simulink library "halout"  (R2021b)
settings: Solver=VariableStepAuto  StartTime=0.0  StopTime=10.0  RelTol=1e-3
undefined symbols (not defined in the file): C_TASK_5MS_S, FALSE, KHAL_CAN1FD1APS3E2E_flg, KHAL_CAN1FD1APS3TxReq_flg, KHAL_CAN1FD1VCU2E2E_flg, KHAL_CAN1FD1VCU2TxReq_flg, KHAL_CAN1FD1VCU3E2E_flg, KHAL_CAN1FD1VCU3TxReq_flg, KHAL_CAN1TxReq_flg, KHAL_CAN1VMCFCM1E2E_flg, KHAL_CAN1VMCFCM1TxReq_flg, KHAL_CAN2TxReq_flg, KHAL_CAN3FD3VCU1toNIDECTxReq_flg, KHAL_CAN3FD3VCU1TxReq_flg, KHAL_CAN3FD3VCU2E2E_flg, KHAL_CAN3FD3VCU2toNIDECE2E_flg, KHAL_CAN3FD3VCU2toNIDECTxReq_flg, KHAL_CAN3FD3VCU2TxReq_flg, KHAL_CAN3TxReq_flg, KHAL_CAN4FD4CE1000E2E_flg, KHAL_CAN4FD4CE1000TxReq_flg, KHAL_CAN4TxReq_flg, KHAL_CAN5TxReq_flg, KHAL_CAN6FD6APS3E2E_flg, KHAL_CAN6FD6APS3TxReq_flg, KHAL_CAN6FD6VCU2E2E_flg, KHAL_CAN6FD6VCU2TxReq_flg, KHAL_CAN6TxReq_flg, ONE_INT, TRUE, ZERO_INT
libraries: FVT_lib x549, simulink x244
(part 17 of 27)

== system halout/HAL_OUT/CAN1/VMC_FCM1_0x172/Byte_13 ==
  FDC_VMC_AngCtrlTqWtGn : Inport
  BitwiseOR : simulink/Logic and Bit Operations/Bitwise Operator  logicop=OR  UseBitMask=off  BitMask=bin2dec('11011001')  BitMaskRealWorld=Stored Integer
  SignalPack : FVT_lib/hal/SignalPack  RightShiftCnt=0  BitMask=2^8-1  LeftShiftCnt=0
  UnitConverter : DataTypeConversion  OutDataTypeStr=uint8  RndMeth=Round
  UnitConverter1 : DataTypeConversion  OutDataTypeStr=uint8  RndMeth=Round
  convert_out : FVT_lib/hal/convert_out  gain=0.4  offset=0
  Byte_13 : Outport
  wires:
  BitwiseOR/1 -> Byte_13/1
  UnitConverter/1 -> BitwiseOR/1
  SignalPack/1 -> UnitConverter/1
  UnitConverter1/1 -> SignalPack/1
  convert_out/1 -> UnitConverter1/1
  FDC_VMC_AngCtrlTqWtGn/1 -> convert_out/1

== system halout/HAL_OUT/CAN1/VMC_FCM1_0x172/Byte_14 ==
  FDC_VMC_DrInpTqBstGn : Inport
  BitwiseOR : simulink/Logic and Bit Operations/Bitwise Operator  logicop=OR  UseBitMask=off  BitMask=bin2dec('11011001')  BitMaskRealWorld=Stored Integer
  SignalPack : FVT_lib/hal/SignalPack  RightShiftCnt=0  BitMask=2^8-1  LeftShiftCnt=0
  UnitConverter : DataTypeConversion  OutDataTypeStr=uint8  RndMeth=Round
  UnitConverter1 : DataTypeConversion  OutDataTypeStr=uint8  RndMeth=Round
  convert_out : FVT_lib/hal/convert_out  gain=0.4  offset=0
  Byte_14 : Outport
  wires:
  BitwiseOR/1 -> Byte_14/1
  UnitConverter/1 -> BitwiseOR/1
  SignalPack/1 -> UnitConverter/1
  UnitConverter1/1 -> SignalPack/1
  convert_out/1 -> UnitConverter1/1
  FDC_VMC_DrInpTqBstGn/1 -> convert_out/1

== system halout/HAL_OUT/CAN1/VMC_FCM1_0x172/Byte_15 ==
  FDC_VMC_DMSMode_Cmd : Inport
  BitwiseOR : simulink/Logic and Bit Operations/Bitwise Operator  logicop=OR  UseBitMask=off  BitMask=bin2dec('11011001')  BitMaskRealWorld=Stored Integer
  SignalPack : FVT_lib/hal/SignalPack  RightShiftCnt=0  BitMask=2^4-1  LeftShiftCnt=0
  UnitConverter : DataTypeConversion  OutDataTypeStr=uint8  RndMeth=Round
  UnitConverter1 : DataTypeConversion  OutDataTypeStr=uint8  RndMeth=Round
  Byte_15 : Outport
  wires:
  BitwiseOR/1 -> Byte_15/1
  UnitConverter/1 -> BitwiseOR/1
  SignalPack/1 -> UnitConverter/1
  UnitConverter1/1 -> SignalPack/1
  FDC_VMC_DMSMode_Cmd/1 -> UnitConverter1/1

== system halout/HAL_OUT/CAN1/VMC_FCM1_0x172/Byte_2 ==
  VMC_FCM_LKA_TOIAct : Inport
  BitwiseOR : simulink/Logic and Bit Operations/Bitwise Operator  logicop=OR  UseBitMask=off  BitMask=bin2dec('11011001')  BitMaskRealWorld=Stored Integer
  SignalPack : FVT_lib/hal/SignalPack  RightShiftCnt=0  BitMask=2^8-1  LeftShiftCnt=0
  UnitConverter : DataTypeConversion  OutDataTypeStr=uint8  RndMeth=Round
  UnitConverter1 : DataTypeConversion  OutDataTypeStr=uint8  RndMeth=Round
  Byte_2 : Outport
  wires:
  BitwiseOR/1 -> Byte_2/1
  UnitConverter/1 -> BitwiseOR/1
  SignalPack/1 -> UnitConverter/1
  UnitConverter1/1 -> SignalPack/1
  VMC_FCM_LKA_TOIAct/1 -> UnitConverter1/1

== system halout/HAL_OUT/CAN1/VMC_FCM1_0x172/Byte_3 ==
  VMC_AEB_VehHoldReq : Inport
  VMC_FCM_LDW_Fault : Inport  Port=2
  VMC_FCM_LDW_Request : Inport  Port=3
  VMC_FCM_LKA_StrToqReq : Inport  Port=4
  VMC_FCM_LKA_TOIFault : Inport  Port=5
  BitwiseOR : simulink/Logic and Bit Operations/Bitwise Operator  logicop=OR  UseBitMask=off  NumInputPorts=5  BitMask=bin2dec('11011001')  BitMaskRealWorld=Stored Integer
  SignalPack : FVT_lib/hal/SignalPack  RightShiftCnt=0  BitMask=2^1-1  LeftShiftCnt=3
  SignalPack1 : FVT_lib/hal/SignalPack  RightShiftCnt=0  BitMask=2^1-1  LeftShiftCnt=5
  SignalPack2 : FVT_lib/hal/SignalPack  RightShiftCnt=0  BitMask=2^2-1  LeftShiftCnt=6
  SignalPack3 : FVT_lib/hal/SignalPack  RightShiftCnt=8  BitMask=2^3-1  LeftShiftCnt=0
  SignalPack4 : FVT_lib/hal/SignalPack  RightShiftCnt=0  BitMask=2^1-1  LeftShiftCnt=4
  UnitConverter{,1..6,8..9} (9 alike) : DataTypeConversion  OutDataTypeStr=uint8  RndMeth=Round
  UnitConverter7 : DataTypeConversion  OutDataTypeStr=uint16  RndMeth=Round
  convert_out : FVT_lib/hal/convert_out  gain=0.008  offset=-8
  Byte_3 : Outport
  wires:
  BitwiseOR/1 -> Byte_3/1
  UnitConverter/1 -> BitwiseOR/1
  SignalPack/1 -> UnitConverter/1
  UnitConverter1/1 -> SignalPack/1
  VMC_AEB_VehHoldReq/1 -> UnitConverter1/1
  UnitConverter2/1 -> BitwiseOR/2
  SignalPack1/1 -> UnitConverter2/1
  UnitConverter3/1 -> SignalPack1/1
  VMC_FCM_LDW_Fault/1 -> UnitConverter3/1
  UnitConverter4/1 -> BitwiseOR/3
  SignalPack2/1 -> UnitConverter4/1
  UnitConverter5/1 -> SignalPack2/1
  VMC_FCM_LDW_Request/1 -> UnitConverter5/1
  UnitConverter6/1 -> BitwiseOR/4
  SignalPack3/1 -> UnitConverter6/1
  UnitConverter7/1 -> SignalPack3/1
  convert_out/1 -> UnitConverter7/1
  VMC_FCM_LKA_StrToqReq/1 -> convert_out/1
  UnitConverter8/1 -> BitwiseOR/5
  SignalPack4/1 -> UnitConverter8/1
  UnitConverter9/1 -> SignalPack4/1
  VMC_FCM_LKA_TOIFault/1 -> UnitConverter9/1

== system halout/HAL_OUT/CAN1/VMC_FCM1_0x172/Byte_4 ==
  VMC_FCM_LKA_StrToqReq : Inport
  BitwiseOR : simulink/Logic and Bit Operations/Bitwise Operator  logicop=OR  UseBitMask=off  BitMask=bin2dec('11011001')  BitMaskRealWorld=Stored Integer
  SignalPack : FVT_lib/hal/SignalPack  RightShiftCnt=0  BitMask=2^8-1  LeftShiftCnt=0
  UnitConverter : DataTypeConversion  OutDataTypeStr=uint8  RndMeth=Round
  UnitConverter1 : DataTypeConversion  OutDataTypeStr=uint16  RndMeth=Round
  convert_out : FVT_lib/hal/convert_out  gain=0.008  offset=-8
  Byte_4 : Outport
  wires:
  BitwiseOR/1 -> Byte_4/1
  UnitConverter/1 -> BitwiseOR/1
  SignalPack/1 -> UnitConverter/1
  UnitConverter1/1 -> SignalPack/1
  convert_out/1 -> UnitConverter1/1
  VMC_FCM_LKA_StrToqReq/1 -> convert_out/1

== system halout/HAL_OUT/CAN1/VMC_FCM1_0x172/Byte_5 ==
  VMC_ACC_RequiredAccel : Inport
  VMC_ACC_VehHoldReq : Inport  Port=2
  VMC_ADAS_AEBReq : Inport  Port=3
  VMC_ADAS_DBSReq : Inport  Port=4
  VMC_ADAS_FaultSta : Inport  Port=5
  BitwiseOR : simulink/Logic and Bit Operations/Bitwise Operator  logicop=OR  UseBitMask=off  NumInputPorts=5  BitMask=bin2dec('11011001')  BitMaskRealWorld=Stored Integer
  SignalPack : FVT_lib/hal/SignalPack  RightShiftCnt=8  BitMask=2^1-1  LeftShiftCnt=0
  SignalPack1 : FVT_lib/hal/SignalPack  RightShiftCnt=0  BitMask=2^1-1  LeftShiftCnt=7
  SignalPack2 : FVT_lib/hal/SignalPack  RightShiftCnt=0  BitMask=2^3-1  LeftShiftCnt=1
  SignalPack3 : FVT_lib/hal/SignalPack  RightShiftCnt=0  BitMask=2^2-1  LeftShiftCnt=5
  SignalPack4 : FVT_lib/hal/SignalPack  RightShiftCnt=0  BitMask=2^1-1  LeftShiftCnt=4
  UnitConverter{,2..9} (9 alike) : DataTypeConversion  OutDataTypeStr=uint8  RndMeth=Round
  UnitConverter1 : DataTypeConversion  OutDataTypeStr=uint16  RndMeth=Round
  convert_out : FVT_lib/hal/convert_out  gain=0.05  offset=-15
  Byte_5 : Outport
  wires:
  BitwiseOR/1 -> Byte_5/1
  UnitConverter/1 -> BitwiseOR/1
  SignalPack/1 -> UnitConverter/1
  UnitConverter1/1 -> SignalPack/1
  convert_out/1 -> UnitConverter1/1
  VMC_ACC_RequiredAccel/1 -> convert_out/1
  UnitConverter2/1 -> BitwiseOR/2
  SignalPack1/1 -> UnitConverter2/1
  UnitConverter3/1 -> SignalPack1/1
  VMC_ACC_VehHoldReq/1 -> UnitConverter3/1
  UnitConverter4/1 -> BitwiseOR/3
  SignalPack2/1 -> UnitConverter4/1
  UnitConverter5/1 -> SignalPack2/1
  VMC_ADAS_AEBReq/1 -> UnitConverter5/1
  UnitConverter6/1 -> BitwiseOR/4
  SignalPack3/1 -> UnitConverter6/1
  UnitConverter7/1 -> SignalPack3/1
  VMC_ADAS_DBSReq/1 -> UnitConverter7/1
  UnitConverter8/1 -> BitwiseOR/5
  SignalPack4/1 -> UnitConverter8/1
  UnitConverter9/1 -> SignalPack4/1
  VMC_ADAS_FaultSta/1 -> UnitConverter9/1

== system halout/HAL_OUT/CAN1/VMC_FCM1_0x172/Byte_6 ==
  VMC_ACC_RequiredAccel : Inport
  BitwiseOR : simulink/Logic and Bit Operations/Bitwise Operator  logicop=OR  UseBitMask=off  BitMask=bin2dec('11011001')  BitMaskRealWorld=Stored Integer
  SignalPack : FVT_lib/hal/SignalPack  RightShiftCnt=0  BitMask=2^8-1  LeftShiftCnt=0
  UnitConverter : DataTypeConversion  OutDataTypeStr=uint8  RndMeth=Round
  UnitConverter1 : DataTypeConversion  OutDataTypeStr=uint16  RndMeth=Round
  convert_out : FVT_lib/hal/convert_out  gain=0.05  offset=-15
  Byte_6 : Outport
  wires:
  BitwiseOR/1 -> Byte_6/1
  UnitConverter/1 -> BitwiseOR/1
  SignalPack/1 -> UnitConverter/1
  UnitConverter1/1 -> SignalPack/1
  convert_out/1 -> UnitConverter1/1
  VMC_ACC_RequiredAccel/1 -> convert_out/1

== system halout/HAL_OUT/CAN1/VMC_FCM1_0x172/Byte_7 ==
  VMC_ACC_ComfortBandUpper : Inport
  VMC_ACC_JerkUpperLInit : Inport  Port=2
  BitwiseOR : simulink/Logic and Bit Operations/Bitwise Operator  logicop=OR  UseBitMask=off  NumInputPorts=2  BitMask=bin2dec('11011001')  BitMaskRealWorld=Stored Integer
  SignalPack : FVT_lib/hal/SignalPack  RightShiftCnt=8  BitMask=2^1-1  LeftShiftCnt=0
  SignalPack1 : FVT_lib/hal/SignalPack  RightShiftCnt=0  BitMask=2^7-1  LeftShiftCnt=1
  UnitConverter : DataTypeConversion  OutDataTypeStr=uint8  RndMeth=Round
  UnitConverter1 : DataTypeConversion  OutDataTypeStr=uint16  RndMeth=Round
  UnitConverter2 : DataTypeConversion  OutDataTypeStr=uint8  RndMeth=Round
  UnitConverter3 : DataTypeConversion  OutDataTypeStr=uint8  RndMeth=Round
  convert_out : FVT_lib/hal/convert_out  gain=0.05  offset=-15
  convert_out1 : FVT_lib/hal/convert_out  gain=0.1  offset=-6
  Byte_7 : Outport
  wires:
  BitwiseOR/1 -> Byte_7/1
  UnitConverter/1 -> BitwiseOR/1
  SignalPack/1 -> UnitConverter/1
  UnitConverter1/1 -> SignalPack/1
  convert_out/1 -> UnitConverter1/1
  VMC_ACC_ComfortBandUpper/1 -> convert_out/1
  UnitConverter2/1 -> BitwiseOR/2
  SignalPack1/1 -> UnitConverter2/1
  UnitConverter3/1 -> SignalPack1/1
  convert_out1/1 -> UnitConverter3/1
  VMC_ACC_JerkUpperLInit/1 -> convert_out1/1

== system halout/HAL_OUT/CAN1/VMC_FCM1_0x172/Byte_8 ==
  VMC_ACC_ComfortBandUpper : Inport
  BitwiseOR : simulink/Logic and Bit Operations/Bitwise Operator  logicop=OR  UseBitMask=off  BitMask=bin2dec('11011001')  BitMaskRealWorld=Stored Integer
  SignalPack : FVT_lib/hal/SignalPack  RightShiftCnt=0  BitMask=2^8-1  LeftShiftCnt=0
  UnitConverter : DataTypeConversion  OutDataTypeStr=uint8  RndMeth=Round
  UnitConverter1 : DataTypeConversion  OutDataTypeStr=uint16  RndMeth=Round
  convert_out : FVT_lib/hal/convert_out  gain=0.05  offset=-15
  Byte_8 : Outport
  wires:
  BitwiseOR/1 -> Byte_8/1
  UnitConverter/1 -> BitwiseOR/1
  SignalPack/1 -> UnitConverter/1
  UnitConverter1/1 -> SignalPack/1
  convert_out/1 -> UnitConverter1/1
  VMC_ACC_ComfortBandUpper/1 -> convert_out/1

== system halout/HAL_OUT/CAN1/VMC_FCM1_0x172/Byte_9 ==
  VMC_ACC_ComfortBandLower : Inport
  VMC_ACC_JerkLowerLInit : Inport  Port=2
  BitwiseOR : simulink/Logic and Bit Operations/Bitwise Operator  logicop=OR  UseBitMask=off  NumInputPorts=2  BitMask=bin2dec('11011001')  BitMaskRealWorld=Stored Integer
  SignalPack : FVT_lib/hal/SignalPack  RightShiftCnt=8  BitMask=2^1-1  LeftShiftCnt=0
  SignalPack1 : FVT_lib/hal/SignalPack  RightShiftCnt=0  BitMask=2^7-1  LeftShiftCnt=1
  UnitConverter : DataTypeConversion  OutDataTypeStr=uint8  RndMeth=Round
  UnitConverter1 : DataTypeConversion  OutDataTypeStr=uint16  RndMeth=Round
  UnitConverter2 : DataTypeConversion  OutDataTypeStr=uint8  RndMeth=Round
  UnitConverter3 : DataTypeConversion  OutDataTypeStr=uint8  RndMeth=Round
  convert_out : FVT_lib/hal/convert_out  gain=0.05  offset=-15
  convert_out1 : FVT_lib/hal/convert_out  gain=0.1  offset=-6
  Byte_9 : Outport
  wires:
  BitwiseOR/1 -> Byte_9/1
  UnitConverter/1 -> BitwiseOR/1
  SignalPack/1 -> UnitConverter/1
  UnitConverter1/1 -> SignalPack/1
  convert_out/1 -> UnitConverter1/1
  VMC_ACC_ComfortBandLower/1 -> convert_out/1
  UnitConverter2/1 -> BitwiseOR/2
  SignalPack1/1 -> UnitConverter2/1
  UnitConverter3/1 -> SignalPack1/1
  convert_out1/1 -> UnitConverter3/1
  VMC_ACC_JerkLowerLInit/1 -> convert_out1/1

== system halout/HAL_OUT/CAN1/VMC_FCM1_0x172/CRC8_IfAction_Tx ==
  CAN_E2E_flg : Inport
  DataID1 : Inport  Port=2
  DataID2 : Inport  Port=3
  RawData : Inport  Port=4
  Data Type Conversion : DataTypeConversion  OutDataTypeStr=uint8
  If : If
  If Action Subsystem : Subsystem  TreatAsAtomicUnit=on
  If Action Subsystem1 : Subsystem  TreatAsAtomicUnit=on
  Merge : Merge
  CRC8 : Outport
  wires:
  If/2 -> If Action Subsystem/Action
  If/1 -> If Action Subsystem1/Action
  CAN_E2E_flg/1 -> [CAN_E2E_flg]
  DataID1/1 -> [DataID1]
  DataID2/1 -> [DataID2]
  RawData/1 -> [RawData]
  [CAN_E2E_flg] -> Data Type Conversion/1
  [DataID1] -> If Action Subsystem1/1(CAN_E2E_ID1)
  [DataID2] -> If Action Subsystem1/2(CAN_E2E_ID2)
  [RawData] -> If Action Subsystem1/3(Byte1)
  [RawData] -> If Action Subsystem/1(Byte1)
  If Action Subsystem1/1(CRC8_E2EResult) -> Merge/1
  If Action Subsystem/1(CRC8_Result) -> Merge/2
  Merge/1 -> CRC8/1
  Data Type Conversion/1 -> If/1

== system halout/HAL_OUT/CAN1/VMC_FCM1_0x172/FDCVMCAngCtrlTqWtGn ==
  FDCVMCAngCtrlTqWtGn : Inport
  Data Type Conversion : DataTypeConversion  OutDataTypeStr=uint8  RndMeth=Round
  convert_out : FVT_lib/hal/convert_out  gain=0.4  offset=0
  CAN1_FDC_VMC_AngCtrlTqWtGn : Outport
  wires:
  Data Type Conversion/1 -> CAN1_FDC_VMC_AngCtrlTqWtGn/1
  convert_out/1 -> Data Type Conversion/1
  FDCVMCAngCtrlTqWtGn/1 -> convert_out/1

== system halout/HAL_OUT/CAN1/VMC_FCM1_0x172/FDCVMCDMSModeCmd ==
  FDCVMCDMSModeCmd : Inport
  Data Type Conversion : DataTypeConversion  OutDataTypeStr=uint8  RndMeth=Round
  CAN1_FDC_VMC_DMSMode_Cmd : Outport
  wires:
  Data Type Conversion/1 -> CAN1_FDC_VMC_DMSMode_Cmd/1
  FDCVMCDMSModeCmd/1 -> Data Type Conversion/1

== system halout/HAL_OUT/CAN1/VMC_FCM1_0x172/FDCVMCDrInpTqBstAct ==
  FDCVMCDrInpTqBstAct : Inport
  Data Type Conversion : DataTypeConversion  OutDataTypeStr=uint8  RndMeth=Round
  CAN1_FDC_VMC_DrInpTqBstAct : Outport
  wires:
  Data Type Conversion/1 -> CAN1_FDC_VMC_DrInpTqBstAct/1
  FDCVMCDrInpTqBstAct/1 -> Data Type Conversion/1

== system halout/HAL_OUT/CAN1/VMC_FCM1_0x172/FDCVMCDrInpTqBstGn ==
  FDCVMCDrInpTqBstGn : Inport
  Data Type Conversion : DataTypeConversion  OutDataTypeStr=uint8  RndMeth=Round
  convert_out : FVT_lib/hal/convert_out  gain=0.4  offset=0
  CAN1_FDC_VMC_DrInpTqBstGn : Outport
  wires:
  Data Type Conversion/1 -> CAN1_FDC_VMC_DrInpTqBstGn/1
  convert_out/1 -> Data Type Conversion/1
  FDCVMCDrInpTqBstGn/1 -> convert_out/1

== system halout/HAL_OUT/CAN1/VMC_FCM1_0x172/FDCVMCMaxAngCtrlOutTqLim ==
  FDCVMCMaxAngCtrlOutTqLim : Inport
  Data Type Conversion : DataTypeConversion  OutDataTypeStr=uint16  RndMeth=Round
  convert_out : FVT_lib/hal/convert_out  gain=0.1  offset=0
  CAN1_FDC_VMC_MaxAngCtrlOutTqLim : Outport
  wires:
  Data Type Conversion/1 -> CAN1_FDC_VMC_MaxAngCtrlOutTqLim/1
  convert_out/1 -> Data Type Conversion/1
  FDCVMCMaxAngCtrlOutTqLim/1 -> convert_out/1

== system halout/HAL_OUT/CAN1/VMC_FCM1_0x172/VMCACCComfortBandLower ==
  VMCACCComfortBandLower : Inport
  Data Type Conversion : DataTypeConversion  OutDataTypeStr=uint16  RndMeth=Round
  convert_out : FVT_lib/hal/convert_out  gain=0.05  offset=-15
  CAN1_VMC_ACC_ComfortBandLower : Outport
  wires:
  Data Type Conversion/1 -> CAN1_VMC_ACC_ComfortBandLower/1
  convert_out/1 -> Data Type Conversion/1
  VMCACCComfortBandLower/1 -> convert_out/1

== system halout/HAL_OUT/CAN1/VMC_FCM1_0x172/VMCACCComfortBandUpper ==
  VMCACCComfortBandUpper : Inport
  Data Type Conversion : DataTypeConversion  OutDataTypeStr=uint16  RndMeth=Round
  convert_out : FVT_lib/hal/convert_out  gain=0.05  offset=-15
  CAN1_VMC_ACC_ComfortBandUpper : Outport
  wires:
  Data Type Conversion/1 -> CAN1_VMC_ACC_ComfortBandUpper/1
  convert_out/1 -> Data Type Conversion/1
  VMCACCComfortBandUpper/1 -> convert_out/1

== system halout/HAL_OUT/CAN1/VMC_FCM1_0x172/VMCACCJerkLowerLInit ==
  VMCACCJerkLowerLInit : Inport
  Data Type Conversion : DataTypeConversion  OutDataTypeStr=uint8  RndMeth=Round
  convert_out : FVT_lib/hal/convert_out  gain=0.1  offset=-6
  CAN1_VMC_ACC_JerkLowerLInit : Outport
  wires:
  Data Type Conversion/1 -> CAN1_VMC_ACC_JerkLowerLInit/1
  convert_out/1 -> Data Type Conversion/1
  VMCACCJerkLowerLInit/1 -> convert_out/1

== system halout/HAL_OUT/CAN1/VMC_FCM1_0x172/VMCACCJerkUpperLInit ==
  VMCACCJerkUpperLInit : Inport
  Data Type Conversion : DataTypeConversion  OutDataTypeStr=uint8  RndMeth=Round
  convert_out : FVT_lib/hal/convert_out  gain=0.1  offset=-6
  CAN1_VMC_ACC_JerkUpperLInit : Outport
  wires:
  Data Type Conversion/1 -> CAN1_VMC_ACC_JerkUpperLInit/1
  convert_out/1 -> Data Type Conversion/1
  VMCACCJerkUpperLInit/1 -> convert_out/1

== system halout/HAL_OUT/CAN1/VMC_FCM1_0x172/VMCACCRequiredAccel ==
  VMCACCRequiredAccel : Inport
  Data Type Conversion : DataTypeConversion  OutDataTypeStr=uint16  RndMeth=Round
  convert_out : FVT_lib/hal/convert_out  gain=0.05  offset=-15
  CAN1_VMC_ACC_RequiredAccel : Outport
  wires:
  Data Type Conversion/1 -> CAN1_VMC_ACC_RequiredAccel/1
  convert_out/1 -> Data Type Conversion/1
  VMCACCRequiredAccel/1 -> convert_out/1

== system halout/HAL_OUT/CAN1/VMC_FCM1_0x172/VMCACCVehHoldReq ==
  VMCACCVehHoldReq : Inport
  Data Type Conversion : DataTypeConversion  OutDataTypeStr=uint8  RndMeth=Round
  CAN1_VMC_ACC_VehHoldReq : Outport
  wires:
  Data Type Conversion/1 -> CAN1_VMC_ACC_VehHoldReq/1
  VMCACCVehHoldReq/1 -> Data Type Conversion/1

== system halout/HAL_OUT/CAN1/VMC_FCM1_0x172/VMCADASACCSta ==
  VMCADASACCSta : Inport
  Data Type Conversion : DataTypeConversion  OutDataTypeStr=uint8  RndMeth=Round
  CAN1_VMC_ADAS_ACC_Sta : Outport
  wires:
  Data Type Conversion/1 -> CAN1_VMC_ADAS_ACC_Sta/1
  VMCADASACCSta/1 -> Data Type Conversion/1

== system halout/HAL_OUT/CAN1/VMC_FCM1_0x172/VMCADASAEBReq ==
  VMCADASAEBReq : Inport
  Data Type Conversion : DataTypeConversion  OutDataTypeStr=uint8  RndMeth=Round
  CAN1_VMC_ADAS_AEBReq : Outport
  wires:
  Data Type Conversion/1 -> CAN1_VMC_ADAS_AEBReq/1
  VMCADASAEBReq/1 -> Data Type Conversion/1

== system halout/HAL_OUT/CAN1/VMC_FCM1_0x172/VMCADASAEBSta ==
  VMCADASAEBSta : Inport
  Data Type Conversion : DataTypeConversion  OutDataTypeStr=uint8  RndMeth=Round
  CAN1_VMC_ADAS_AEB_Sta : Outport
  wires:
  Data Type Conversion/1 -> CAN1_VMC_ADAS_AEB_Sta/1
  VMCADASAEBSta/1 -> Data Type Conversion/1

== system halout/HAL_OUT/CAN1/VMC_FCM1_0x172/VMCADASDBSReq ==
  VMCADASDBSReq : Inport
  Data Type Conversion : DataTypeConversion  OutDataTypeStr=uint8  RndMeth=Round
  CAN1_VMC_ADAS_DBSReq : Outport
  wires:
  Data Type Conversion/1 -> CAN1_VMC_ADAS_DBSReq/1
  VMCADASDBSReq/1 -> Data Type Conversion/1

== system halout/HAL_OUT/CAN1/VMC_FCM1_0x172/VMCADASFaultSta ==
  VMCADASFaultSta : Inport
  Data Type Conversion : DataTypeConversion  OutDataTypeStr=uint8  RndMeth=Round
  CAN1_VMC_ADAS_FaultSta : Outport
  wires:
  Data Type Conversion/1 -> CAN1_VMC_ADAS_FaultSta/1
  VMCADASFaultSta/1 -> Data Type Conversion/1

== system halout/HAL_OUT/CAN1/VMC_FCM1_0x172/VMCAEBVehHoldReq ==
  VMCAEBVehHoldReq : Inport
  Data Type Conversion : DataTypeConversion  OutDataTypeStr=uint8  RndMeth=Round
  CAN1_VMC_AEB_VehHoldReq : Outport
  wires:
  Data Type Conversion/1 -> CAN1_VMC_AEB_VehHoldReq/1
  VMCAEBVehHoldReq/1 -> Data Type Conversion/1

== system halout/HAL_OUT/CAN1/VMC_FCM1_0x172/VMCFCM1Checksum ==
  VMCFCM1Checksum : Inport
  Data Type Conversion : DataTypeConversion  OutDataTypeStr=uint8  RndMeth=Round
  CAN1_VMC_FCM1_Checksum : Outport
  wires:
  Data Type Conversion/1 -> CAN1_VMC_FCM1_Checksum/1
  VMCFCM1Checksum/1 -> Data Type Conversion/1

== system halout/HAL_OUT/CAN1/VMC_FCM1_0x172/VMCFCM1LifeCount ==
  VMCFCM1LifeCount : Inport
  Data Type Conversion : DataTypeConversion  OutDataTypeStr=uint8  RndMeth=Round
  CAN1_VMC_FCM1_LifeCount : Outport
  wires:
  Data Type Conversion/1 -> CAN1_VMC_FCM1_LifeCount/1
  VMCFCM1LifeCount/1 -> Data Type Conversion/1

== system halout/HAL_OUT/CAN1/VMC_FCM1_0x172/VMCFCMLDWFault ==
  VMCFCMLDWFault : Inport
  Data Type Conversion : DataTypeConversion  OutDataTypeStr=uint8  RndMeth=Round
  CAN1_VMC_FCM_LDW_Fault : Outport
  wires:
  Data Type Conversion/1 -> CAN1_VMC_FCM_LDW_Fault/1
  VMCFCMLDWFault/1 -> Data Type Conversion/1

== system halout/HAL_OUT/CAN1/VMC_FCM1_0x172/VMCFCMLDWRequest ==
  VMCFCMLDWRequest : Inport
  Data Type Conversion : DataTypeConversion  OutDataTypeStr=uint8  RndMeth=Round
  CAN1_VMC_FCM_LDW_Request : Outport
  wires:
  Data Type Conversion/1 -> CAN1_VMC_FCM_LDW_Request/1
  VMCFCMLDWRequest/1 -> Data Type Conversion/1

== system halout/HAL_OUT/CAN1/VMC_FCM1_0x172/VMCFCMLKAStrToqReq ==
  VMCFCMLKAStrToqReq : Inport
  Data Type Conversion : DataTypeConversion  OutDataTypeStr=uint16  RndMeth=Round
  convert_out : FVT_lib/hal/convert_out  gain=0.008  offset=-8
  CAN1_VMC_FCM_LKA_StrToqReq : Outport
  wires:
  Data Type Conversion/1 -> CAN1_VMC_FCM_LKA_StrToqReq/1
  convert_out/1 -> Data Type Conversion/1
  VMCFCMLKAStrToqReq/1 -> convert_out/1

== system halout/HAL_OUT/CAN1/VMC_FCM1_0x172/VMCFCMLKATOIAct ==
  VMCFCMLKATOIAct : Inport
  Data Type Conversion : DataTypeConversion  OutDataTypeStr=uint8  RndMeth=Round
  CAN1_VMC_FCM_LKA_TOIAct : Outport
  wires:
  Data Type Conversion/1 -> CAN1_VMC_FCM_LKA_TOIAct/1
  VMCFCMLKATOIAct/1 -> Data Type Conversion/1

== system halout/HAL_OUT/CAN1/VMC_FCM1_0x172/VMCFCMLKATOIFault ==
  VMCFCMLKATOIFault : Inport
  Data Type Conversion : DataTypeConversion  OutDataTypeStr=uint8  RndMeth=Round
  CAN1_VMC_FCM_LKA_TOIFault : Outport
  wires:
  Data Type Conversion/1 -> CAN1_VMC_FCM_LKA_TOIFault/1
  VMCFCMLKATOIFault/1 -> Data Type Conversion/1

== system halout/HAL_OUT/CAN2/FD2_C20_0_0x210/APSExitCondition ==
  APSExitCondition : Inport
  Data Type Conversion : DataTypeConversion  OutDataTypeStr=uint8  RndMeth=Round
  CAN2_APS_ExitCondition : Outport
  wires:
  Data Type Conversion/1 -> CAN2_APS_ExitCondition/1
  APSExitCondition/1 -> Data Type Conversion/1

== system halout/HAL_OUT/CAN2/FD2_C20_0_0x210/APSRQDisplay ==
  APSRQDisplay : Inport
  Data Type Conversion : DataTypeConversion  OutDataTypeStr=uint8  RndMeth=Round
  CAN2_APS_RQ_Display : Outport
  wires:
  Data Type Conversion/1 -> CAN2_APS_RQ_Display/1
  APSRQDisplay/1 -> Data Type Conversion/1

== system halout/HAL_OUT/CAN2/FD2_C20_0_0x210/APSSWVer ==
  APSSWVer : Inport
  Data Type Conversion : DataTypeConversion  OutDataTypeStr=uint8  RndMeth=Round
  CAN2_APS_SW_Ver : Outport
  wires:
  Data Type Conversion/1 -> CAN2_APS_SW_Ver/1
  APSSWVer/1 -> Data Type Conversion/1

== system halout/HAL_OUT/CAN2/FD2_C20_0_0x210/APSStaSystem ==
  APSStaSystem : Inport
  Data Type Conversion : DataTypeConversion  OutDataTypeStr=uint8  RndMeth=Round
  CAN2_APS_Sta_System : Outport
  wires:
  Data Type Conversion/1 -> CAN2_APS_Sta_System/1
  APSStaSystem/1 -> Data Type Conversion/1

== system halout/HAL_OUT/CAN2/FD2_C20_0_0x210/CAASSta ==
  CAASSta : Inport
  Data Type Conversion : DataTypeConversion  OutDataTypeStr=uint8  RndMeth=Round
  CAN2_CAAS_Sta : Outport
  wires:
  Data Type Conversion/1 -> CAN2_CAAS_Sta/1
  CAASSta/1 -> Data Type Conversion/1

== system halout/HAL_OUT/CAN2/FD2_C20_0_0x210/DISCDISCTargetSpd ==
  DISCDISCTargetSpd : Inport
  Data Type Conversion : DataTypeConversion  OutDataTypeStr=uint16  RndMeth=Round
  convert_out : FVT_lib/hal/convert_out  gain=0.125  offset=0
  CAN2_DISC_DISCTargetSpd : Outport
  wires:
  Data Type Conversion/1 -> CAN2_DISC_DISCTargetSpd/1
  convert_out/1 -> Data Type Conversion/1
  DISCDISCTargetSpd/1 -> convert_out/1

== system halout/HAL_OUT/CAN2/FD2_C20_0_0x210/FDCVCURegenLimIndSta ==
  FDCVCURegenLimIndSta : Inport
  Data Type Conversion : DataTypeConversion  OutDataTypeStr=uint8  RndMeth=Round
  CAN2_FDC_VCU_RegenLimInd_Sta : Outport
  wires:
  Data Type Conversion/1 -> CAN2_FDC_VCU_RegenLimInd_Sta/1
  FDCVCURegenLimIndSta/1 -> Data Type Conversion/1

== system halout/HAL_OUT/CAN2/FD2_C20_0_0x210/FDCVCURegenModeSta ==
  FDCVCURegenModeSta : Inport
  Data Type Conversion : DataTypeConversion  OutDataTypeStr=uint8  RndMeth=Round
  CAN2_FDC_VCU_RegenMode_Sta : Outport
  wires:
  Data Type Conversion/1 -> CAN2_FDC_VCU_RegenMode_Sta/1
  FDCVCURegenModeSta/1 -> Data Type Conversion/1

== system halout/HAL_OUT/CAN2/FD2_C20_0_0x210/FDCVCUSmartEcoSpdLimSta ==
  FDCVCUSmartEcoSpdLimSta : Inport
  Data Type Conversion : DataTypeConversion  OutDataTypeStr=uint8  RndMeth=Round
  CAN2_FDC_VCU_SmartEcoSpdLim_Sta : Outport
  wires:
  Data Type Conversion/1 -> CAN2_FDC_VCU_SmartEcoSpdLim_Sta/1
  FDCVCUSmartEcoSpdLimSta/1 -> Data Type Conversion/1

== system halout/HAL_OUT/CAN2/FD2_C20_0_0x210/FDCVCUSmartEcoSta ==
  FDCVCUSmartEcoSta : Inport
  Data Type Conversion : DataTypeConversion  OutDataTypeStr=uint8  RndMeth=Round
  CAN2_FDC_VCU_SmartEco_Sta : Outport
  wires:
  Data Type Conversion/1 -> CAN2_FDC_VCU_SmartEco_Sta/1
  FDCVCUSmartEcoSta/1 -> Data Type Conversion/1

== system halout/HAL_OUT/CAN2/FD2_C20_0_0x210/FDCVMCSetSpdDispSta ==
  FDCVMCSetSpdDispSta : Inport
  Data Type Conversion : DataTypeConversion  OutDataTypeStr=uint8  RndMeth=Round
  CAN2_FDC_VMC_SetSpdDisp_Sta : Outport
  wires:
  Data Type Conversion/1 -> CAN2_FDC_VMC_SetSpdDisp_Sta/1
  FDCVMCSetSpdDispSta/1 -> Data Type Conversion/1

== system halout/HAL_OUT/CAN2/FD2_C20_0_0x210/FDCVMCSetSpdSta ==
  FDCVMCSetSpdSta : Inport
  Data Type Conversion : DataTypeConversion  OutDataTypeStr=uint8  RndMeth=Round
  CAN2_FDC_VMC_SetSpd_Sta : Outport
  wires:
  Data Type Conversion/1 -> CAN2_FDC_VMC_SetSpd_Sta/1
  FDCVMCSetSpdSta/1 -> Data Type Conversion/1

== system halout/HAL_OUT/CAN2/FD2_C20_0_0x210/FDCVMCSpdCtrlModeSta ==
  FDCVMCSpdCtrlModeSta : Inport
  Data Type Conversion : DataTypeConversion  OutDataTypeStr=uint8  RndMeth=Round
  CAN2_FDC_VMC_SpdCtrlMode_Sta : Outport
  wires:
  Data Type Conversion/1 -> CAN2_FDC_VMC_SpdCtrlMode_Sta/1
  FDCVMCSpdCtrlModeSta/1 -> Data Type Conversion/1

== system halout/HAL_OUT/CAN2/FD2_C20_0_0x210/FDCVMCSpdCtrlSta ==
  FDCVMCSpdCtrlSta : Inport
  Data Type Conversion : DataTypeConversion  OutDataTypeStr=uint8  RndMeth=Round
  CAN2_FDC_VMC_SpdCtrl_Sta : Outport
  wires:
  Data Type Conversion/1 -> CAN2_FDC_VMC_SpdCtrl_Sta/1
  FDCVMCSpdCtrlSta/1 -> Data Type Conversion/1

== system halout/HAL_OUT/CAN2/FD2_C20_0_0x210/PASAFCL ==
  PASAFCL : Inport
  Data Type Conversion : DataTypeConversion  OutDataTypeStr=uint8  RndMeth=Round
  CAN2_PAS_A_FCL : Outport
  wires:
  Data Type Conversion/1 -> CAN2_PAS_A_FCL/1
  PASAFCL/1 -> Data Type Conversion/1

== system halout/HAL_OUT/CAN2/FD2_C20_0_0x210/PASAFCR ==
  PASAFCR : Inport
  Data Type Conversion : DataTypeConversion  OutDataTypeStr=uint8  RndMeth=Round
  CAN2_PAS_A_FCR : Outport
  wires:
  Data Type Conversion/1 -> CAN2_PAS_A_FCR/1
  PASAFCR/1 -> Data Type Conversion/1

== system halout/HAL_OUT/CAN2/FD2_C20_0_0x210/PASAFML ==
  PASAFML : Inport
  Data Type Conversion : DataTypeConversion  OutDataTypeStr=uint8  RndMeth=Round
  CAN2_PAS_A_FML : Outport
  wires:
  Data Type Conversion/1 -> CAN2_PAS_A_FML/1
  PASAFML/1 -> Data Type Conversion/1

== system halout/HAL_OUT/CAN2/FD2_C20_0_0x210/PASAFMR ==
  PASAFMR : Inport
  Data Type Conversion : DataTypeConversion  OutDataTypeStr=uint8  RndMeth=Round
  CAN2_PAS_A_FMR : Outport
  wires:
  Data Type Conversion/1 -> CAN2_PAS_A_FMR/1
  PASAFMR/1 -> Data Type Conversion/1

== system halout/HAL_OUT/CAN2/FD2_C20_0_0x210/PASARCL ==
  PASARCL : Inport
  Data Type Conversion : DataTypeConversion  OutDataTypeStr=uint8  RndMeth=Round
  CAN2_PAS_A_RCL : Outport
  wires:
  Data Type Conversion/1 -> CAN2_PAS_A_RCL/1
  PASARCL/1 -> Data Type Conversion/1

== system halout/HAL_OUT/CAN2/FD2_C20_0_0x210/PASARCR ==
  PASARCR : Inport
  Data Type Conversion : DataTypeConversion  OutDataTypeStr=uint8  RndMeth=Round
  CAN2_PAS_A_RCR : Outport
  wires:
  Data Type Conversion/1 -> CAN2_PAS_A_RCR/1
  PASARCR/1 -> Data Type Conversion/1

== system halout/HAL_OUT/CAN2/FD2_C20_0_0x210/PASARML ==
  PASARML : Inport
  Data Type Conversion : DataTypeConversion  OutDataTypeStr=uint8  RndMeth=Round
  CAN2_PAS_A_RML : Outport
  wires:
  Data Type Conversion/1 -> CAN2_PAS_A_RML/1
  PASARML/1 -> Data Type Conversion/1

== system halout/HAL_OUT/CAN2/FD2_C20_0_0x210/PASARMR ==
  PASARMR : Inport
  Data Type Conversion : DataTypeConversion  OutDataTypeStr=uint8  RndMeth=Round
  CAN2_PAS_A_RMR : Outport
  wires:
  Data Type Conversion/1 -> CAN2_PAS_A_RMR/1
  PASARMR/1 -> Data Type Conversion/1

== system halout/HAL_OUT/CAN2/FD2_C20_0_0x210/PASChime ==
  PASChime : Inport
  Data Type Conversion : DataTypeConversion  OutDataTypeStr=uint8  RndMeth=Round
  CAN2_PAS_Chime : Outport
  wires:
  Data Type Conversion/1 -> CAN2_PAS_Chime/1
  PASChime/1 -> Data Type Conversion/1

== system halout/HAL_OUT/CAN2/FD2_C20_0_0x210/PASDFCL ==
  PASDFCL : Inport
  Data Type Conversion : DataTypeConversion  OutDataTypeStr=uint8  RndMeth=Round
  CAN2_PAS_D_FCL : Outport
  wires:
  Data Type Conversion/1 -> CAN2_PAS_D_FCL/1
  PASDFCL/1 -> Data Type Conversion/1

== system halout/HAL_OUT/CAN2/FD2_C20_0_0x210/PASDFCR ==
  PASDFCR : Inport
  Data Type Conversion : DataTypeConversion  OutDataTypeStr=uint8  RndMeth=Round
  CAN2_PAS_D_FCR : Outport
  wires:
  Data Type Conversion/1 -> CAN2_PAS_D_FCR/1
  PASDFCR/1 -> Data Type Conversion/1

== system halout/HAL_OUT/CAN2/FD2_C20_0_0x210/PASDFML ==
  PASDFML : Inport
  Data Type Conversion : DataTypeConversion  OutDataTypeStr=uint8  RndMeth=Round
  CAN2_PAS_D_FML : Outport
  wires:
  Data Type Conversion/1 -> CAN2_PAS_D_FML/1
  PASDFML/1 -> Data Type Conversion/1

== system halout/HAL_OUT/CAN2/FD2_C20_0_0x210/PASDFMR ==
  PASDFMR : Inport
  Data Type Conversion : DataTypeConversion  OutDataTypeStr=uint8  RndMeth=Round
  CAN2_PAS_D_FMR : Outport
  wires:
  Data Type Conversion/1 -> CAN2_PAS_D_FMR/1
  PASDFMR/1 -> Data Type Conversion/1

== system halout/HAL_OUT/CAN2/FD2_C20_0_0x210/PASDRCL ==
  PASDRCL : Inport
  Data Type Conversion : DataTypeConversion  OutDataTypeStr=uint8  RndMeth=Round
  CAN2_PAS_D_RCL : Outport
  wires:
  Data Type Conversion/1 -> CAN2_PAS_D_RCL/1
  PASDRCL/1 -> Data Type Conversion/1

== system halout/HAL_OUT/CAN2/FD2_C20_0_0x210/PASDRCR ==
  PASDRCR : Inport
  Data Type Conversion : DataTypeConversion  OutDataTypeStr=uint8  RndMeth=Round
  CAN2_PAS_D_RCR : Outport
  wires:
  Data Type Conversion/1 -> CAN2_PAS_D_RCR/1
  PASDRCR/1 -> Data Type Conversion/1

== system halout/HAL_OUT/CAN2/FD2_C20_0_0x210/PASDRML ==
  PASDRML : Inport
  Data Type Conversion : DataTypeConversion  OutDataTypeStr=uint8  RndMeth=Round
  CAN2_PAS_D_RML : Outport
  wires:
  Data Type Conversion/1 -> CAN2_PAS_D_RML/1
  PASDRML/1 -> Data Type Conversion/1

== system halout/HAL_OUT/CAN2/FD2_C20_0_0x210/PASDRMR ==
  PASDRMR : Inport
  Data Type Conversion : DataTypeConversion  OutDataTypeStr=uint8  RndMeth=Round
  CAN2_PAS_D_RMR : Outport
  wires:
  Data Type Conversion/1 -> CAN2_PAS_D_RMR/1
  PASDRMR/1 -> Data Type Conversion/1

== system halout/HAL_OUT/CAN2/FD2_C20_0_0x210/PASSNSRLayout ==
  PASSNSRLayout : Inport
  Data Type Conversion : DataTypeConversion  OutDataTypeStr=uint8  RndMeth=Round
  CAN2_PAS_SNSR_Layout : Outport
  wires:
  Data Type Conversion/1 -> CAN2_PAS_SNSR_Layout/1
  PASSNSRLayout/1 -> Data Type Conversion/1

== system halout/HAL_OUT/CAN2/FD2_C20_0_0x210/USSStaFCL ==
  USSStaFCL : Inport
  Data Type Conversion : DataTypeConversion  OutDataTypeStr=uint8  RndMeth=Round
  CAN2_USS_Sta_FCL : Outport
  wires:
  Data Type Conversion/1 -> CAN2_USS_Sta_FCL/1
  USSStaFCL/1 -> Data Type Conversion/1

== system halout/HAL_OUT/CAN2/FD2_C20_0_0x210/USSStaFCR ==
  USSStaFCR : Inport
  Data Type Conversion : DataTypeConversion  OutDataTypeStr=uint8  RndMeth=Round
  CAN2_USS_Sta_FCR : Outport
  wires:
  Data Type Conversion/1 -> CAN2_USS_Sta_FCR/1
  USSStaFCR/1 -> Data Type Conversion/1

== system halout/HAL_OUT/CAN2/FD2_C20_0_0x210/USSStaFLL ==
  USSStaFLL : Inport
  Data Type Conversion : DataTypeConversion  OutDataTypeStr=uint8  RndMeth=Round
  CAN2_USS_Sta_FLL : Outport
  wires:
  Data Type Conversion/1 -> CAN2_USS_Sta_FLL/1
  USSStaFLL/1 -> Data Type Conversion/1

== system halout/HAL_OUT/CAN2/FD2_C20_0_0x210/USSStaFLR ==
  USSStaFLR : Inport
  Data Type Conversion : DataTypeConversion  OutDataTypeStr=uint8  RndMeth=Round
  CAN2_USS_Sta_FLR : Outport
  wires:
  Data Type Conversion/1 -> CAN2_USS_Sta_FLR/1
  USSStaFLR/1 -> Data Type Conversion/1

== system halout/HAL_OUT/CAN2/FD2_C20_0_0x210/USSStaFML ==
  USSStaFML : Inport
  Data Type Conversion : DataTypeConversion  OutDataTypeStr=uint8  RndMeth=Round
  CAN2_USS_Sta_FML : Outport
  wires:
  Data Type Conversion/1 -> CAN2_USS_Sta_FML/1
  USSStaFML/1 -> Data Type Conversion/1

== system halout/HAL_OUT/CAN2/FD2_C20_0_0x210/USSStaFMR ==
  USSStaFMR : Inport
  Data Type Conversion : DataTypeConversion  OutDataTypeStr=uint8  RndMeth=Round
  CAN2_USS_Sta_FMR : Outport
  wires:
  Data Type Conversion/1 -> CAN2_USS_Sta_FMR/1
  USSStaFMR/1 -> Data Type Conversion/1

== system halout/HAL_OUT/CAN2/FD2_C20_0_0x210/USSStaRCL ==
  USSStaRCL : Inport
  Data Type Conversion : DataTypeConversion  OutDataTypeStr=uint8  RndMeth=Round
  CAN2_USS_Sta_RCL : Outport
  wires:
  Data Type Conversion/1 -> CAN2_USS_Sta_RCL/1
  USSStaRCL/1 -> Data Type Conversion/1

== system halout/HAL_OUT/CAN2/FD2_C20_0_0x210/USSStaRCR ==
  USSStaRCR : Inport
  Data Type Conversion : DataTypeConversion  OutDataTypeStr=uint8  RndMeth=Round
  CAN2_USS_Sta_RCR : Outport
  wires:
  Data Type Conversion/1 -> CAN2_USS_Sta_RCR/1
  USSStaRCR/1 -> Data Type Conversion/1

== system halout/HAL_OUT/CAN2/FD2_C20_0_0x210/USSStaRLL ==
  USSStaRLL : Inport
  Data Type Conversion : DataTypeConversion  OutDataTypeStr=uint8  RndMeth=Round
  CAN2_USS_Sta_RLL : Outport
  wires:
  Data Type Conversion/1 -> CAN2_USS_Sta_RLL/1
  USSStaRLL/1 -> Data Type Conversion/1

== system halout/HAL_OUT/CAN2/FD2_C20_0_0x210/USSStaRLR ==
  USSStaRLR : Inport
  Data Type Conversion : DataTypeConversion  OutDataTypeStr=uint8  RndMeth=Round
  CAN2_USS_Sta_RLR : Outport
  wires:
  Data Type Conversion/1 -> CAN2_USS_Sta_RLR/1
  USSStaRLR/1 -> Data Type Conversion/1

== system halout/HAL_OUT/CAN2/FD2_C20_0_0x210/USSStaRML ==
  USSStaRML : Inport
  Data Type Conversion : DataTypeConversion  OutDataTypeStr=uint8  RndMeth=Round
  CAN2_USS_Sta_RML : Outport
  wires:
  Data Type Conversion/1 -> CAN2_USS_Sta_RML/1
  USSStaRML/1 -> Data Type Conversion/1

== system halout/HAL_OUT/CAN2/FD2_C20_0_0x210/USSStaRMR ==
  USSStaRMR : Inport
  Data Type Conversion : DataTypeConversion  OutDataTypeStr=uint8  RndMeth=Round
  CAN2_USS_Sta_RMR : Outport
  wires:
  Data Type Conversion/1 -> CAN2_USS_Sta_RMR/1
  USSStaRMR/1 -> Data Type Conversion/1

== system halout/HAL_OUT/CAN2/FD2_C20_0_0x210/VMCVCUCCCrlSta ==
  VMCVCUCCCrlSta : Inport
  Data Type Conversion : DataTypeConversion  OutDataTypeStr=uint8  RndMeth=Round
  CAN2_VMC_VCU_CC_Crl_Sta : Outport
  wires:
  Data Type Conversion/1 -> CAN2_VMC_VCU_CC_Crl_Sta/1
  VMCVCUCCCrlSta/1 -> Data Type Conversion/1

== system halout/HAL_OUT/CAN2/FD2_C20_0_0x210/VMCVCUMSACrlSta ==
  VMCVCUMSACrlSta : Inport
  Data Type Conversion : DataTypeConversion  OutDataTypeStr=uint8  RndMeth=Round
  CAN2_VMC_VCU_MSA_Crl_Sta : Outport
  wires:
  Data Type Conversion/1 -> CAN2_VMC_VCU_MSA_Crl_Sta/1
  VMCVCUMSACrlSta/1 -> Data Type Conversion/1

== system halout/HAL_OUT/CAN2/FD2_CE100_0_0x117/APMDoorControlSta ==
  APMDoorControlSta : Inport
  Data Type Conversion : DataTypeConversion  OutDataTypeStr=uint8  RndMeth=Round
  CAN2_APMDoorControlSta : Outport
  wires:
  Data Type Conversion/1 -> CAN2_APMDoorControlSta/1
  APMDoorControlSta/1 -> Data Type Conversion/1

== system halout/HAL_OUT/CAN2/FD2_CE100_0_0x117/ActAPSPosn ==
  ActAPSPosn : Inport
  Data Type Conversion : DataTypeConversion  OutDataTypeStr=uint8  RndMeth=Round
  convert_out : FVT_lib/hal/convert_out  gain=0.394  offset=0
  CAN2_ActAPSPosn : Outport
  wires:
  Data Type Conversion/1 -> CAN2_ActAPSPosn/1
  convert_out/1 -> Data Type Conversion/1
  ActAPSPosn/1 -> convert_out/1

== system halout/HAL_OUT/CAN2/FD2_CE100_0_0x117/AllDoorSW ==
  AllDoorSW : Inport
  Data Type Conversion : DataTypeConversion  OutDataTypeStr=uint8  RndMeth=Round
  CAN2_AllDoorSW : Outport
  wires:
  Data Type Conversion/1 -> CAN2_AllDoorSW/1
  AllDoorSW/1 -> Data Type Conversion/1

== system halout/HAL_OUT/CAN2/FD2_CE100_0_0x117/AntitheftSta ==
  AntitheftSta : Inport
  Data Type Conversion : DataTypeConversion  OutDataTypeStr=uint8  RndMeth=Round
  CAN2_AntitheftSta : Outport
  wires:
  Data Type Conversion/1 -> CAN2_AntitheftSta/1
  AntitheftSta/1 -> Data Type Conversion/1

== system halout/HAL_OUT/CAN2/FD2_CE100_0_0x117/BCMDoorLockSta ==
  BCMDoorLockSta : Inport
  Data Type Conversion : DataTypeConversion  OutDataTypeStr=uint8  RndMeth=Round
  CAN2_BCM_DoorLock_Sta : Outport
  wires:
  Data Type Conversion/1 -> CAN2_BCM_DoorLock_Sta/1
  BCMDoorLockSta/1 -> Data Type Conversion/1

== system halout/HAL_OUT/CAN2/FD2_CE100_0_0x117/BrakeLamp ==
  BrakeLamp : Inport
  Data Type Conversion : DataTypeConversion  OutDataTypeStr=uint8  RndMeth=Round
  CAN2_BrakeLamp : Outport
  wires:
  Data Type Conversion/1 -> CAN2_BrakeLamp/1
  BrakeLamp/1 -> Data Type Conversion/1

== system halout/HAL_OUT/CAN2/FD2_CE100_0_0x117/CCCrlSta ==
  CCCrlSta : Inport
  Data Type Conversion : DataTypeConversion  OutDataTypeStr=uint8  RndMeth=Round
  CAN2_CC_Crl_Sta : Outport
  wires:
  Data Type Conversion/1 -> CAN2_CC_Crl_Sta/1
  CCCrlSta/1 -> Data Type Conversion/1

== system halout/HAL_OUT/CAN2/FD2_CE100_0_0x117/CCMSASpdWar ==
  CCMSASpdWar : Inport
  Data Type Conversion : DataTypeConversion  OutDataTypeStr=uint8  RndMeth=Round
  CAN2_CCMSA_SpdWar : Outport
  wires:
  Data Type Conversion/1 -> CAN2_CCMSA_SpdWar/1
  CCMSASpdWar/1 -> Data Type Conversion/1

== system halout/HAL_OUT/CAN2/FD2_CE100_0_0x117/CCUACLampSts ==
  CCUACLampSts : Inport
  Data Type Conversion : DataTypeConversion  OutDataTypeStr=uint8  RndMeth=Round
  CAN2_CCU_ACLampSts : Outport
  wires:
  Data Type Conversion/1 -> CAN2_CCU_ACLampSts/1
  CCUACLampSts/1 -> Data Type Conversion/1

== system halout/HAL_OUT/CAN2/FD2_CE100_0_0x117/CCUACMaxLampSts ==
  CCUACMaxLampSts : Inport
  Data Type Conversion : DataTypeConversion  OutDataTypeStr=uint8  RndMeth=Round
  CAN2_CCU_ACMaxLampSts : Outport
  wires:
  Data Type Conversion/1 -> CAN2_CCU_ACMaxLampSts/1
  CCUACMaxLampSts/1 -> Data Type Conversion/1

== system halout/HAL_OUT/CAN2/FD2_CE100_0_0x117/CCUAutoLampSts ==
  CCUAutoLampSts : Inport
  Data Type Conversion : DataTypeConversion  OutDataTypeStr=uint8  RndMeth=Round
  CAN2_CCU_AutoLampSts : Outport
  wires:
  Data Type Conversion/1 -> CAN2_CCU_AutoLampSts/1
  CCUAutoLampSts/1 -> Data Type Conversion/1

== system halout/HAL_OUT/CAN2/FD2_CE100_0_0x117/CCUAutoMidLampSts ==
  CCUAutoMidLampSts : Inport
  Data Type Conversion : DataTypeConversion  OutDataTypeStr=uint8  RndMeth=Round
  CAN2_CCU_AutoMidLampSts : Outport
  wires:
  Data Type Conversion/1 -> CAN2_CCU_AutoMidLampSts/1
  CCUAutoMidLampSts/1 -> Data Type Conversion/1

== system halout/HAL_OUT/CAN2/FD2_CE100_0_0x117/CCUDispalyRequest ==
  CCUDispalyRequest : Inport
  Data Type Conversion : DataTypeConversion  OutDataTypeStr=uint8  RndMeth=Round
  CAN2_CCU_Dispaly_Request : Outport
  wires:
  Data Type Conversion/1 -> CAN2_CCU_Dispaly_Request/1
  CCUDispalyRequest/1 -> Data Type Conversion/1

== system halout/HAL_OUT/CAN2/FD2_CE100_0_0x117/CCUEcoSts ==
  CCUEcoSts : Inport
  Data Type Conversion : DataTypeConversion  OutDataTypeStr=uint8  RndMeth=Round
  CAN2_CCU_EcoSts : Outport
  wires:
  Data Type Conversion/1 -> CAN2_CCU_EcoSts/1
  CCUEcoSts/1 -> Data Type Conversion/1

== system halout/HAL_OUT/CAN2/FD2_CE100_0_0x117/CCUFrtOnOffLampSts ==
  CCUFrtOnOffLampSts : Inport
  Data Type Conversion : DataTypeConversion  OutDataTypeStr=uint8  RndMeth=Round
  CAN2_CCU_FrtOnOffLampSts : Outport
  wires:
  Data Type Conversion/1 -> CAN2_CCU_FrtOnOffLampSts/1
  CCUFrtOnOffLampSts/1 -> Data Type Conversion/1

== system halout/HAL_OUT/CAN2/FD2_CE100_0_0x117/CCURrOnOffLampSts ==
  CCURrOnOffLampSts : Inport
  Data Type Conversion : DataTypeConversion  OutDataTypeStr=uint8  RndMeth=Round
  CAN2_CCU_RrOnOffLampSts : Outport
  wires:
  Data Type Conversion/1 -> CAN2_CCU_RrOnOffLampSts/1
  CCURrOnOffLampSts/1 -> Data Type Conversion/1

== system halout/HAL_OUT/CAN2/FD2_CE100_0_0x117/CCUSyncLampSts ==
  CCUSyncLampSts : Inport
  Data Type Conversion : DataTypeConversion  OutDataTypeStr=uint8  RndMeth=Round
  CAN2_CCU_SyncLampSts : Outport
  wires:
  Data Type Conversion/1 -> CAN2_CCU_SyncLampSts/1
  CCUSyncLampSts/1 -> Data Type Conversion/1

== system halout/HAL_OUT/CAN2/FD2_CE100_0_0x117/CoastDwModeStaChk ==
  CoastDwModeStaChk : Inport
  Data Type Conversion : DataTypeConversion  OutDataTypeStr=uint8  RndMeth=Round
  CAN2_CoastDwModeStaChk : Outport
  wires:
  Data Type Conversion/1 -> CAN2_CoastDwModeStaChk/1
  CoastDwModeStaChk/1 -> Data Type Conversion/1

== system halout/HAL_OUT/CAN2/FD2_CE100_0_0x117/CreepSWSta ==
  CreepSWSta : Inport
  Data Type Conversion : DataTypeConversion  OutDataTypeStr=uint8  RndMeth=Round
  CAN2_CreepSW_Sta : Outport
  wires:
  Data Type Conversion/1 -> CAN2_CreepSW_Sta/1
  CreepSWSta/1 -> Data Type Conversion/1

== system halout/HAL_OUT/CAN2/FD2_CE100_0_0x117/DISCButtSta ==
  DISCButtSta : Inport
  Data Type Conversion : DataTypeConversion  OutDataTypeStr=uint8  RndMeth=Round
  CAN2_DISC_ButtSta : Outport
  wires:
  Data Type Conversion/1 -> CAN2_DISC_ButtSta/1
  DISCButtSta/1 -> Data Type Conversion/1

== system halout/HAL_OUT/CAN2/FD2_CE100_0_0x117/DISCSta ==
  DISCSta : Inport
  Data Type Conversion : DataTypeConversion  OutDataTypeStr=uint8  RndMeth=Round
  CAN2_DISC_Sta : Outport
  wires:
  Data Type Conversion/1 -> CAN2_DISC_Sta/1
  DISCSta/1 -> Data Type Conversion/1

== system halout/HAL_OUT/CAN2/FD2_CE100_0_0x117/DemoModeStaChk ==
  DemoModeStaChk : Inport
  Data Type Conversion : DataTypeConversion  OutDataTypeStr=uint8  RndMeth=Round
  CAN2_DemoModeStaChk : Outport
  wires:
  Data Type Conversion/1 -> CAN2_DemoModeStaChk/1
  DemoModeStaChk/1 -> Data Type Conversion/1

== system halout/HAL_OUT/CAN2/FD2_CE100_0_0x117/Dimmer ==
  Dimmer : Inport
  Data Type Conversion : DataTypeConversion  OutDataTypeStr=uint8  RndMeth=Round
  CAN2_Dimmer : Outport
  wires:
  Data Type Conversion/1 -> CAN2_Dimmer/1
  Dimmer/1 -> Data Type Conversion/1

== system halout/HAL_OUT/CAN2/FD2_CE100_0_0x117/DimmerEN ==
  DimmerEN : Inport
  Data Type Conversion : DataTypeConversion  OutDataTypeStr=uint8  RndMeth=Round
  CAN2_DimmerEN : Outport
  wires:
  Data Type Conversion/1 -> CAN2_DimmerEN/1
  DimmerEN/1 -> Data Type Conversion/1

== system halout/HAL_OUT/CAN2/FD2_CE100_0_0x117/DisengagePFail ==
  DisengagePFail : Inport
  Data Type Conversion : DataTypeConversion  OutDataTypeStr=uint8  RndMeth=Round
  CAN2_DisengageP_Fail : Outport
  wires:
  Data Type Conversion/1 -> CAN2_DisengageP_Fail/1
  DisengagePFail/1 -> Data Type Conversion/1

== system halout/HAL_OUT/CAN2/FD2_CE100_0_0x117/DoorLockIND ==
  DoorLockIND : Inport
  Data Type Conversion : DataTypeConversion  OutDataTypeStr=uint8  RndMeth=Round
  CAN2_DoorLockIND : Outport
  wires:
  Data Type Conversion/1 -> CAN2_DoorLockIND/1
  DoorLockIND/1 -> Data Type Conversion/1

== system halout/HAL_OUT/CAN2/FD2_CE100_0_0x117/DrDoorSW ==
  DrDoorSW : Inport
  Data Type Conversion : DataTypeConversion  OutDataTypeStr=uint8  RndMeth=Round
  CAN2_DrDoorSW : Outport
  wires:
  Data Type Conversion/1 -> CAN2_DrDoorSW/1
  DrDoorSW/1 -> Data Type Conversion/1

== system halout/HAL_OUT/CAN2/FD2_CE100_0_0x117/DrSeatSta ==
  DrSeatSta : Inport
  Data Type Conversion : DataTypeConversion  OutDataTypeStr=uint8  RndMeth=Round
  CAN2_Dr_SeatSta : Outport
  wires:
  Data Type Conversion/1 -> CAN2_Dr_SeatSta/1
  DrSeatSta/1 -> Data Type Conversion/1

== system halout/HAL_OUT/CAN2/FD2_CE100_0_0x117/DynoModeStaChk ==
  DynoModeStaChk : Inport
  Data Type Conversion : DataTypeConversion  OutDataTypeStr=uint8  RndMeth=Round
  CAN2_DynoModeStaChk : Outport
  wires:
  Data Type Conversion/1 -> CAN2_DynoModeStaChk/1
  DynoModeStaChk/1 -> Data Type Conversion/1

== system halout/HAL_OUT/CAN2/FD2_CE100_0_0x117/EDriveSysErrAccPedalErr ==
  EDriveSysErrAccPedalErr : Inport
  Data Type Conversion : DataTypeConversion  OutDataTypeStr=uint8  RndMeth=Round
  CAN2_EDriveSysErr_AccPedalErr : Outport
  wires:
  Data Type Conversion/1 -> CAN2_EDriveSysErr_AccPedalErr/1
  EDriveSysErrAccPedalErr/1 -> Data Type Conversion/1

== system halout/HAL_OUT/CAN2/FD2_CE100_0_0x117/EDriveSysErrMCUErr ==
  EDriveSysErrMCUErr : Inport
  Data Type Conversion : DataTypeConversion  OutDataTypeStr=uint8  RndMeth=Round
  CAN2_EDriveSysErr_MCUErr : Outport
  wires:
  Data Type Conversion/1 -> CAN2_EDriveSysErr_MCUErr/1
  EDriveSysErrMCUErr/1 -> Data Type Conversion/1

== system halout/HAL_OUT/CAN2/FD2_CE100_0_0x117/EDriveSysErrShifterErr ==
  EDriveSysErrShifterErr : Inport
  Data Type Conversion : DataTypeConversion  OutDataTypeStr=uint8  RndMeth=Round
  CAN2_EDriveSysErr_ShifterErr : Outport
  wires:
  Data Type Conversion/1 -> CAN2_EDriveSysErr_ShifterErr/1
  EDriveSysErrShifterErr/1 -> Data Type Conversion/1

== system halout/HAL_OUT/CAN2/FD2_CE100_0_0x117/EDriveSysErrVCUErr ==
  EDriveSysErrVCUErr : Inport
  Data Type Conversion : DataTypeConversion  OutDataTypeStr=uint8  RndMeth=Round
  CAN2_EDriveSysErr_VCUErr : Outport
  wires:
  Data Type Conversion/1 -> CAN2_EDriveSysErr_VCUErr/1
  EDriveSysErrVCUErr/1 -> Data Type Conversion/1

== system halout/HAL_OUT/CAN2/FD2_CE100_0_0x117/EVDriveMode ==
  EVDriveMode : Inport
  Data Type Conversion : DataTypeConversion  OutDataTypeStr=uint8  RndMeth=Round
  CAN2_EVDriveMode : Outport
  wires:
  Data Type Conversion/1 -> CAN2_EVDriveMode/1
  EVDriveMode/1 -> Data Type Conversion/1

== system halout/HAL_OUT/CAN2/FD2_CE100_0_0x117/EngAGSCloseSta ==
  EngAGSCloseSta : Inport
  Data Type Conversion : DataTypeConversion  OutDataTypeStr=uint8  RndMeth=Round
  CAN2_Eng_AGSCloseSta : Outport
  wires:
  Data Type Conversion/1 -> CAN2_Eng_AGSCloseSta/1
  EngAGSCloseSta/1 -> Data Type Conversion/1

== system halout/HAL_OUT/CAN2/FD2_CE100_0_0x117/EngActvDmpDisabSta ==
  EngActvDmpDisabSta : Inport
  Data Type Conversion : DataTypeConversion  OutDataTypeStr=uint8  RndMeth=Round
  CAN2_Eng_ActvDmpDisabSta : Outport
  wires:
  Data Type Conversion/1 -> CAN2_Eng_ActvDmpDisabSta/1
  EngActvDmpDisabSta/1 -> Data Type Conversion/1

== system halout/HAL_OUT/CAN2/FD2_CE100_0_0x117/EngCoastDwSta ==
  EngCoastDwSta : Inport
  Data Type Conversion : DataTypeConversion  OutDataTypeStr=uint8  RndMeth=Round
  CAN2_Eng_CoastDwSta : Outport
  wires:
  Data Type Conversion/1 -> CAN2_Eng_CoastDwSta/1
  EngCoastDwSta/1 -> Data Type Conversion/1

== system halout/HAL_OUT/CAN2/FD2_CE100_0_0x117/EngPwrLockSta ==
  EngPwrLockSta : Inport
  Data Type Conversion : DataTypeConversion  OutDataTypeStr=uint8  RndMeth=Round
  CAN2_Eng_PwrLockSta : Outport
  wires:
  Data Type Conversion/1 -> CAN2_Eng_PwrLockSta/1
  EngPwrLockSta/1 -> Data Type Conversion/1

== system halout/HAL_OUT/CAN2/FD2_CE100_0_0x117/EngagePFail ==
  EngagePFail : Inport
  Data Type Conversion : DataTypeConversion  OutDataTypeStr=uint8  RndMeth=Round
  CAN2_EngageP_Fail : Outport
  wires:
  Data Type Conversion/1 -> CAN2_EngageP_Fail/1
  EngagePFail/1 -> Data Type Conversion/1

== system halout/HAL_OUT/CAN2/FD2_CE100_0_0x117/FDABSWarning ==
  FDABSWarning : Inport
  Data Type Conversion : DataTypeConversion  OutDataTypeStr=uint8  RndMeth=Round
  CAN2_FD_ABS_Warning : Outport
  wires:
  Data Type Conversion/1 -> CAN2_FD_ABS_Warning/1
  FDABSWarning/1 -> Data Type Conversion/1

== system halout/HAL_OUT/CAN2/FD2_CE100_0_0x117/FDAGSCmd ==
  FDAGSCmd : Inport
  Data Type Conversion : DataTypeConversion  OutDataTypeStr=uint8  RndMeth=Round
  CAN2_FD_AGS_Cmd : Outport
  wires:
  Data Type Conversion/1 -> CAN2_FD_AGS_Cmd/1
  FDAGSCmd/1 -> Data Type Conversion/1

== system halout/HAL_OUT/CAN2/FD2_CE100_0_0x117/FDBatteryChargeWarning ==
  FDBatteryChargeWarning : Inport
  Data Type Conversion : DataTypeConversion  OutDataTypeStr=uint8  RndMeth=Round
  CAN2_FD_Battery_Charge_Warning : Outport
  wires:
  Data Type Conversion/1 -> CAN2_FD_Battery_Charge_Warning/1
  FDBatteryChargeWarning/1 -> Data Type Conversion/1

== system halout/HAL_OUT/CAN2/FD2_CE100_0_0x117/FDCBCMAutoWipHSpdENSta ==
  FDCBCMAutoWipHSpdENSta : Inport
  Data Type Conversion : DataTypeConversion  OutDataTypeStr=uint8  RndMeth=Round
  CAN2_FDC_BCM_AutoWipHSpdEN_Sta : Outport
  wires:
  Data Type Conversion/1 -> CAN2_FDC_BCM_AutoWipHSpdEN_Sta/1
  FDCBCMAutoWipHSpdENSta/1 -> Data Type Conversion/1

== system halout/HAL_OUT/CAN2/FD2_CE100_0_0x117/FDCBCMHMIKey1FuncSta ==
  FDCBCMHMIKey1FuncSta : Inport
  Data Type Conversion : DataTypeConversion  OutDataTypeStr=uint8  RndMeth=Round
  CAN2_FDC_BCM_HMIKey1Func_Sta : Outport
  wires:
  Data Type Conversion/1 -> CAN2_FDC_BCM_HMIKey1Func_Sta/1
  FDCBCMHMIKey1FuncSta/1 -> Data Type Conversion/1
